simulink model "Cockcroft_walton"  (R2013a)
settings: Solver=ode23  SolverMode=SingleTasking  StartTime=0.0  StopTime=1  RelTol=1e-3
libraries: powerlib x9
settings Model: CovHTMLOptions=-sRT=1 -aTS=1 -bRG=1 -bTC=1 -hTR=0 -nFC=0 -scm=1 -bcm=1 -xEv=0  CovSaveSingleToWorkspaceVar=off  Creator=ASUS  LastModifiedBy=SUJIT
settings DataIOCC: SignalLoggingSaveFormat=ModelDataLogs
settings OptimizationCC: BlockReduction=off  BooleanDataType=off
settings DebuggingCC: SaveWithParameterizedLinksMsg=none  SignalResolutionControl=TryResolveAllWithWarning  SolverPrmCheckMsg=none  MultiTaskDSMMsg=warning  MultiTaskCondExecSysMsg=none  StrictBusMsg=None
settings HardwareCC: TargetUnknown=on
settings RTWCC: IncludeERTFirstTime=on

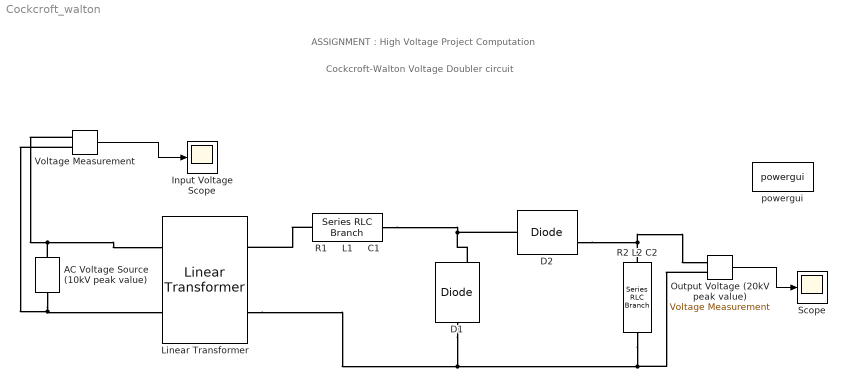
== system Cockcroft_walton ==
  note: Cockcroft-Walton Voltage Doubler circuit
  note: ASSIGNMENT : High Voltage Project Computation
  AC Voltage Source (10kV peak value) : powerlib/Electrical Sources/AC Voltage Source  Amplitude=10000  Phase=0  Frequency=50  SampleTime=0  Measurements=None
  D1 : powerlib/Power Electronics/Diode  Ron=0.001  Lon=0  Vf=55  IC=0  UseSnubber=off  Rs=5000  Cs=250e-12  Measurements=on
  D2 : powerlib/Power Electronics/Diode  Ron=0.001  Lon=0  Vf=55  IC=0  UseSnubber=off  Rs=5000  Cs=500e-13  Measurements=on
  Input Voltage Scope : Scope
      settings: YMin=-12500  YMax=12500
  Linear Transformer : powerlib/Elements/Linear Transformer  LConnTagsString=a|b  RConnTagsString=A|B  UNITS=pu  NominalPower=[ 250e6 60 ]  winding1=[7.35e+05 0.002 0.08]  winding2=[7.35e+05 0.002 0.08]  ThreeWindings=off  winding3=[3.15e+05 0.002 0.08]  RmLm=[500.02 500]  Measurements=None  DataType=off
  Output Voltage (20kV peak value) : powerlib/Measurements/Voltage Measurement  PhasorSimulation=off  OutputType=Complex  PSBequivalent=0
  R1     L1     C1 : powerlib/Elements/Series RLC Branch  LConnTagsString=__new0  RConnTagsString=__new0  BranchType=RLC  Resistance=1000  Inductance=0.001  SetiL0=off  InitialCurrent=0  Capacitance=1e-7  Setx0=off  InitialVoltage=0  Measurements=None
  R2 L2 C2 : powerlib/Elements/Series RLC Branch  LConnTagsString=__new0  RConnTagsString=__new0  BranchType=RLC  Resistance=1000  Inductance=0.001  SetiL0=off  InitialCurrent=0  Capacitance=1e-7  Setx0=off  InitialVoltage=0  Measurements=Branch voltage
  Scope : Scope
      settings: YMin=4000  YMax=20000
  Voltage Measurement : powerlib/Measurements/Voltage Measurement  PhasorSimulation=off  OutputType=Complex  PSBequivalent=0
  powergui : powerlib/powergui  Priority=1  SimulationMode=Continuous  SolverType=Tustin  SampleTime=50e-6  frequency=60  SPID=off  DisableSnubberDevices=off  DisableRonSwitches=off  DisableVfSwitches=off  SwTol=0  Interpol=off  DisplayEquations=off  frequencyindice=50  Pbase=100e6  ErrMax=1e-4  Iterations=50  UnitsV=kV  UnitsW=MW  FunctionMessages=off  echomessages=off  HookPort=off  EnableUseOfTLC=off  x0status=blocks  RestoreLinks=warning  ResistiveCurrentMeasurement=off  Frange=[0:2:500]  Ylog=off  Xlog=on  ShowGrid=off  save=off  variable=ZData  ZoomFFT=off  StartTime=0.0  cycles=1  DisplayStyle=1  fundamental=60  FreqAxis=off  MaxFrequency=1000  frequencyindicesteady=1  RmsSteady=2  display=off  Ts=0  methode=off
  wires:
  Voltage Measurement/1 -> Input Voltage Scope/1
  Output Voltage (20kV peak value)/1 -> Scope/1
  connections:
  D1/LConn1 -- Output Voltage (20kV peak value)/LConn2 -- R2 L2 C2/RConn1 -- Linear Transformer/RConn2
  R2 L2 C2/LConn1 -- D2/RConn1 -- Output Voltage (20kV peak value)/LConn1
  D1/RConn1 -- R1     L1     C1/RConn1 -- D2/LConn1
  AC Voltage Source (10kV peak value)/LConn1 -- Voltage Measurement/LConn2 -- Linear Transformer/LConn2
  AC Voltage Source (10kV peak value)/RConn1 -- Voltage Measurement/LConn1 -- Linear Transformer/LConn1
  R1     L1     C1/LConn1 -- Linear Transformer/RConn1
